simulink model "chap5_2sim"  (Simulink 6.3)
settings: Solver=ode45  StartTime=0.0  StopTime=100  FixedStep=0.001  RelTol=1e-3
libraries: simulink_extras x1
settings Model: LastModifiedBy=Administrator  ExtModeTrigMode=oneshot  ExtModeArmWhenConnect=off  StrictBusMsg=None
settings DataIOCC: LimitDataPoints=off  SignalLoggingName=sigsOut
settings OptimizationCC: BooleanDataType=off
settings DebuggingCC: SolverPrmCheckMsg=none
settings HardwareCC: TargetUnknown=on

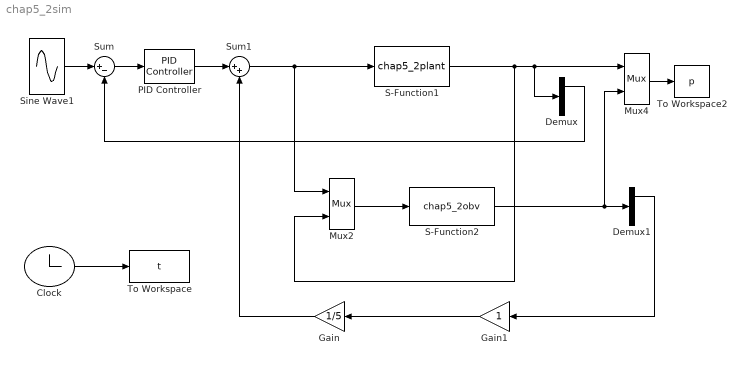
== system chap5_2sim ==
  Clock : Clock
  Demux : Demux  Outputs=2
  Demux1 : Demux  Outputs=2
  Gain : Gain  Orientation=left  Gain=1/5  SaturateOnIntegerOverflow=on
  Gain1 : Gain  Orientation=left  SaturateOnIntegerOverflow=on
  Mux2 : Mux  Inputs=2
  Mux4 : Mux  Inputs=2
  PID Controller : simulink_extras/Additional Linear/PID Controller  P=100  I=0  D=10
  S-Function1 : S-Function  FunctionName=chap5_2plant
  S-Function2 : S-Function  FunctionName=chap5_2obv
  Sine Wave1 : Sin  SampleTime=0
  Sum : Sum  Inputs=|+-  SaturateOnIntegerOverflow=on
  Sum1 : Sum  Inputs=|++  SaturateOnIntegerOverflow=on
  To Workspace : ToWorkspace  VariableName=t  SampleTime=-1  SaveFormat=Array
  To Workspace2 : ToWorkspace  VariableName=p  SampleTime=-1  SaveFormat=Array
  wires:
  S-Function1/1 -> Mux2/2, Mux4/1, Demux/1
  Clock/1 -> To Workspace/1
  Mux4/1 -> To Workspace2/1
  S-Function2/1 -> Mux4/2, Demux1/1
  Mux2/1 -> S-Function2/1
  Demux1/1 -> Gain1/1
  PID Controller/1 -> Sum1/1
  Sum1/1 -> S-Function1/1, Mux2/1
  Gain/1 -> Sum1/2
  Gain1/1 -> Gain/1
  Sum/1 -> PID Controller/1
  Sine Wave1/1 -> Sum/1
  Demux/1 -> Sum/2
